simulink model "Lab11"  (R2021a)
settings: Solver=VariableStepAuto  StartTime=0.0  StopTime=10.0  RelTol=1e-3
undefined symbols (not defined in the file): b1, b2, b3, F_1, F_2, F_3, k1, k2, k3, m1, m2, m3, time_F_1, time_F_2, time_F_3, x1_0, x2_0, x3_0
settings Model: Creator=Alex  LastModifiedBy=Alex

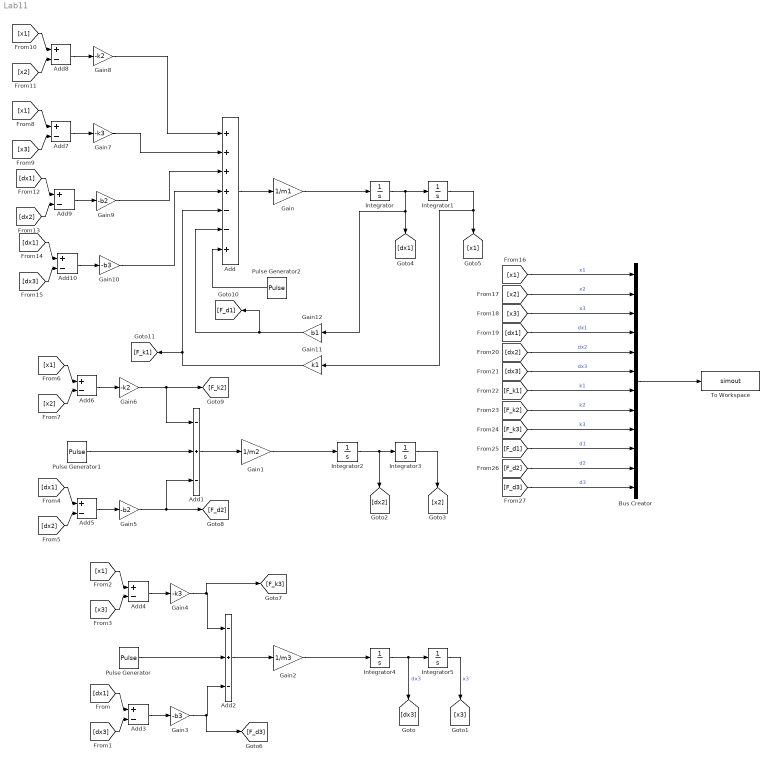
== system Lab11 ==
  Add : Sum  Inputs=++++--+
  Add1 : Sum  Inputs=-+-
  Add{3..10} (8 alike) : Sum  Inputs=+-
  Add2 : Sum  Inputs=-+-
  Bus Creator : BusCreator  Inputs=12
  Gain : Gain  Gain=1/m1
  Gain1 : Gain  Gain=1/m2
  Gain10 : Gain  Gain=-b3
  Gain11 : Gain  Gain=k1
  Gain12 : Gain  Gain=b1
  Gain2 : Gain  Gain=1/m3
  Gain3 : Gain  Gain=-b3
  Gain4 : Gain  Gain=-k3
  Gain5 : Gain  Gain=-b2
  Gain6 : Gain  Gain=-k2
  Gain7 : Gain  Gain=-k3
  Gain8 : Gain  Gain=-k2
  Gain9 : Gain  Gain=-b2
  Integrator : Integrator
  Integrator1 : Integrator  InitialCondition=x1_0
  Integrator2 : Integrator
  Integrator3 : Integrator  InitialCondition=x2_0
  Integrator4 : Integrator
  Integrator5 : Integrator  InitialCondition=x3_0
  Pulse Generator : DiscretePulseGenerator  PulseType=Time based  Amplitude=F_3  Period=t  PulseWidth=100 * time_F_3 / t
  Pulse Generator1 : DiscretePulseGenerator  PulseType=Time based  Amplitude=F_2  Period=t  PulseWidth=100 * time_F_2 / t
  Pulse Generator2 : DiscretePulseGenerator  PulseType=Time based  Amplitude=F_1  Period=t  PulseWidth=100*time_F_1 / t
  To Workspace : ToWorkspace  VariableName=simout  SaveFormat=Timeseries  SampleTime=-1
  wires:
  Gain/1 -> Integrator/1
  Integrator/1 -> Gain12/1, [dx1], Integrator1/1
  Add/1 -> Gain/1
  Gain1/1 -> Integrator2/1
  Integrator2/1 -> [dx2], Integrator3/1
  Add1/1 -> Gain1/1
  Gain2/1 -> Integrator4/1
  Add2/1 -> Gain2/1
  Integrator4/1 -> [dx3], Integrator5/1  "dx3"
  Integrator5/1 -> [x3]  "x3"
  [dx1] -> Add3/1
  [dx3] -> Add3/2
  Gain3/1 -> [F_d3], Add2/3
  Add3/1 -> Gain3/1
  [x1] -> Add4/1
  [x3] -> Add4/2
  Add4/1 -> Gain4/1
  Gain4/1 -> [F_k3], Add2/1
  Pulse Generator/1 -> Add2/2
  Pulse Generator1/1 -> Add1/2
  Add5/1 -> Gain5/1
  [x2] -> Add6/2
  Add6/1 -> Gain6/1
  [dx1] -> Add5/1
  [dx2] -> Add5/2
  Gain5/1 -> Add1/3, [F_d2]
  [x1] -> Add6/1
  Gain6/1 -> [F_k2], Add1/1
  Integrator3/1 -> [x2]
  Integrator1/1 -> Gain11/1, [x1]
  [x3] -> Add7/2
  Add7/1 -> Gain7/1
  [x1] -> Add7/1
  [x2] -> Add8/2
  Add8/1 -> Gain8/1
  Gain8/1 -> Add/1
  [x1] -> Add8/1
  Gain7/1 -> Add/2
  [dx2] -> Add9/2
  Add9/1 -> Gain9/1
  [dx1] -> Add9/1
  Gain9/1 -> Add/3
  [dx3] -> Add10/2
  Add10/1 -> Gain10/1
  Gain10/1 -> Add/4
  [dx1] -> Add10/1
  Gain11/1 -> [F_k1], Add/5
  Gain12/1 -> [F_d1], Add/6
  Pulse Generator2/1 -> Add/7
  Bus Creator/1 -> To Workspace/1
  [x1] -> Bus Creator/1  "x1"
  [x2] -> Bus Creator/2  "x2"
  [x3] -> Bus Creator/3  "x3"
  [dx1] -> Bus Creator/4  "dx1"
  [dx2] -> Bus Creator/5  "dx2"
  [dx3] -> Bus Creator/6  "dx3"
  [F_d1] -> Bus Creator/10  "d1"
  [F_k1] -> Bus Creator/7  "k1"
  [F_k3] -> Bus Creator/9  "k3"
  [F_d3] -> Bus Creator/12  "d3"
  [F_k2] -> Bus Creator/8  "k2"
  [F_d2] -> Bus Creator/11  "d2"
